simulink model "playback_data_example"  (R2016a)
settings: Solver=FixedStepDiscrete  SolverMode=SingleTasking  StartTime=76  StopTime=110  FixedStep=sample_time  RelTol=1e-3
values from neighbouring files (symbols this model uses):
  sample_time = 0.0005    [ElmoIncremental.m]
undefined symbols (not defined in the file or in its folder): control_start_time
libraries: simulink x1
settings Model: Creator=wmartin  LastModifiedBy=wmartin
settings SolverCC: EnableConcurrentExecution=on
settings DataIOCC: MaxDataPoints=1000000000  SaveFormat=StructureWithTime  SignalLogging=off  DSMLogging=off  VisualizeSimOutput=off
settings OptimizationCC: BlockReduction=off  OptimizeBlockIOStorage=off  BufferReuse=off  GlobalBufferReuse=off  ExpressionFolding=off  ExpressionDepthLimit=2147483647  LocalBlockOutputs=off  SimCompilerOptimization=on
settings DebuggingCC: UnderspecifiedInitializationDetection=Classic  MergeDetectMultiDrivingBlocksExec=none  SolverPrmCheckMsg=warning  StateNameClashWarn=warning
settings HardwareCC: ProdBitPerPointer=32  ProdLargestAtomicFloat=None  ProdWordSize=32  ProdLongLongMode=on  ProdHWDeviceType=Generic->32-bit x86 compatible
settings ModelReferenceCC: UpdateModelReferenceTargets=IfOutOfDate  ModelReferenceNumInstancesAllowed=Single  ModelReferenceMinAlgLoopOccurrences=on  PropagateSignalLabelsOutOfModel=off
settings RTWCC: SystemTargetFile=slrt.tlc  TemplateMakefile=slrt_default_tmf  Description=Simulink Real-Time  RTWVerbose=off  RTWCompilerOptimization=on
settings CodeAppCC: MaxIdLength=256
settings TargetCC: CodeReplacementLibrary=XPC_BLAS  ParMdlRefBuildCompliant=on  ConcurrentExecutionCompliant=on  MatFileLogging=on  MATLABClassNameForMDSCustomization=xpcAperiodicCustomization
settings ConfigComp: CovModelRefEnable=Off  CovSFcnEnable=off

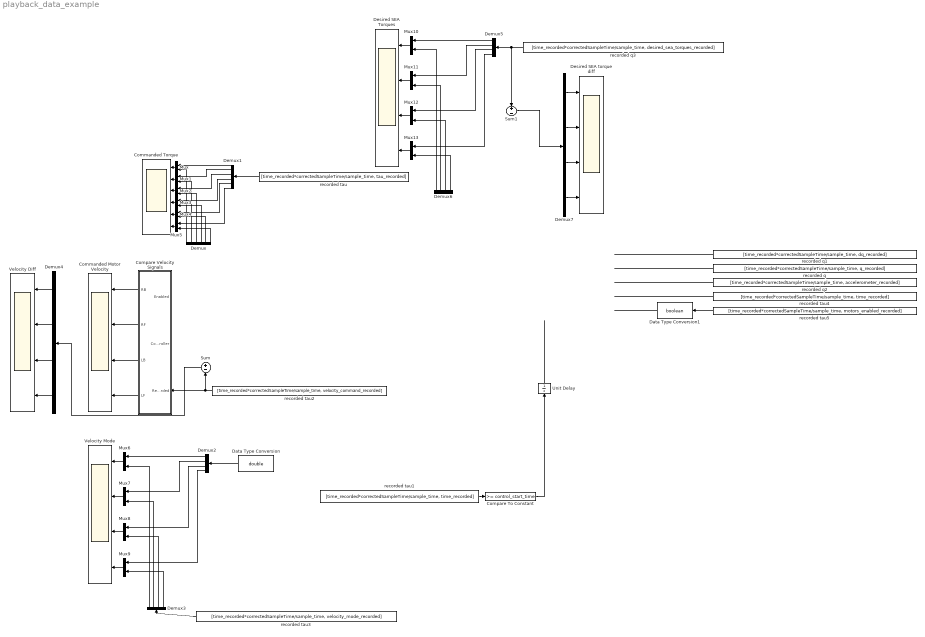
== system playback_data_example ==
  Commanded Motor Velocity : Scope  NumInputPorts=4
  Commanded Torque : Scope  NumInputPorts=6
  Compare To Constant : simulink/Logic and Bit Operations/Compare To Constant  relop=>=  const=control_start_time  OutDataTypeStr=boolean
  Compare Velocity Signals : Subsystem
  Data Type Conversion : DataTypeConversion  OutDataTypeStr=double
  Data Type Conversion1 : DataTypeConversion  OutDataTypeStr=boolean
  Demux : Demux  Outputs=6
  Demux1 : Demux  Outputs=6
  Demux{2..7} (6 alike) : Demux
  Desired SEA Torques : Scope  NumInputPorts=4
  Desired SEA torque diff : Scope  NumInputPorts=4
  Mux{,1..13} (14 alike) : Mux  Inputs=2
  Sum : Sum  Inputs=+-
  Sum1 : Sum  Inputs=+-
  Unit Delay : UnitDelay  SampleTime=-1
  Velocity Diff : Scope  NumInputPorts=4
  Velocity Mode : Scope  NumInputPorts=4
  recorded q : FromWorkspace  VariableName=[time_recorded*correctedSampleTime/sample_time, q_recorded]  OutDataTypeStr=double  SampleTime=sample_time  OutputAfterFinalValue=Holding final value
  recorded q1 : FromWorkspace  VariableName=[time_recorded*correctedSampleTime/sample_time, dq_recorded]  OutDataTypeStr=double  SampleTime=sample_time  OutputAfterFinalValue=Holding final value
  recorded q2 : FromWorkspace  VariableName=[time_recorded*correctedSampleTime/sample_time, accelerometer_recorded]  OutDataTypeStr=double  SampleTime=sample_time  OutputAfterFinalValue=Holding final value
  recorded q3 : FromWorkspace  VariableName=[time_recorded*correctedSampleTime/sample_time, desired_sea_torques_recorded]  OutDataTypeStr=double  SampleTime=sample_time  OutputAfterFinalValue=Holding final value
  recorded tau : FromWorkspace  VariableName=[time_recorded*correctedSampleTime/sample_time, tau_recorded]  OutDataTypeStr=double  SampleTime=sample_time  Interpolate=off  OutputAfterFinalValue=Holding final value
  recorded tau1 : FromWorkspace  VariableName=[time_recorded*correctedSampleTime/sample_time, time_recorded]  OutDataTypeStr=double  SampleTime=sample_time  OutputAfterFinalValue=Holding final value
  recorded tau2 : FromWorkspace  VariableName=[time_recorded*correctedSampleTime/sample_time, velocity_command_recorded]  OutDataTypeStr=double  SampleTime=sample_time  Interpolate=off  OutputAfterFinalValue=Holding final value
  recorded tau3 : FromWorkspace  VariableName=[time_recorded*correctedSampleTime/sample_time, velocity_mode_recorded]  OutDataTypeStr=double  SampleTime=sample_time  Interpolate=off  OutputAfterFinalValue=Holding final value
  recorded tau4 : FromWorkspace  VariableName=[time_recorded*correctedSampleTime/sample_time, time_recorded]  OutDataTypeStr=double  SampleTime=sample_time  OutputAfterFinalValue=Holding final value
  recorded tau5 : FromWorkspace  VariableName=[time_recorded*correctedSampleTime/sample_time, motors_enabled_recorded]  OutDataTypeStr=double  SampleTime=sample_time  OutputAfterFinalValue=Holding final value
  wires:
  recorded tau1/1 -> Compare To Constant/1
  Compare To Constant/1 -> Unit Delay/1
  Unit Delay/1 -> ?
  ? -> Demux/1
  recorded tau/1 -> Demux1/1
  Mux/1 -> Commanded Torque/1
  Mux1/1 -> Commanded Torque/2
  Mux2/1 -> Commanded Torque/3
  Mux3/1 -> Commanded Torque/4
  Mux4/1 -> Commanded Torque/5
  Mux5/1 -> Commanded Torque/6
  Demux1/1 -> Mux/1
  Demux/1 -> Mux/2
  Demux1/2 -> Mux1/1
  Demux1/3 -> Mux2/1
  Demux1/4 -> Mux3/1
  Demux1/5 -> Mux4/1
  Demux1/6 -> Mux5/1
  Demux/2 -> Mux1/2
  Demux/3 -> Mux2/2
  Demux/4 -> Mux3/2
  Demux/5 -> Mux4/2
  Demux/6 -> Mux5/2
  Compare Velocity Signals/1(RB) -> Commanded Motor Velocity/1
  Compare Velocity Signals/2(RF) -> Commanded Motor Velocity/2
  Compare Velocity Signals/3(LB) -> Commanded Motor Velocity/3
  Compare Velocity Signals/4(LF) -> Commanded Motor Velocity/4
  ? -> Compare Velocity Signals/1(Enabled), Data Type Conversion/1
  recorded tau2/1 -> Sum/2, Compare Velocity Signals/3(Recorded)
  Mux6/1 -> Velocity Mode/1
  Mux7/1 -> Velocity Mode/2
  Mux8/1 -> Velocity Mode/3
  Mux9/1 -> Velocity Mode/4
  Demux2/2 -> Mux7/1
  Demux2/3 -> Mux8/1
  Demux2/4 -> Mux9/1
  recorded tau3/1 -> Demux3/1
  Demux3/1 -> Mux6/2
  Demux3/2 -> Mux7/2
  Demux3/3 -> Mux8/2
  Demux3/4 -> Mux9/2
  Data Type Conversion/1 -> Demux2/1
  Demux2/1 -> Mux6/1
  ? -> Sum/1, Compare Velocity Signals/2(Controller)
  Sum/1 -> Demux4/1
  Demux4/4 -> Velocity Diff/4
  Demux4/3 -> Velocity Diff/3
  Demux4/2 -> Velocity Diff/2
  Demux4/1 -> Velocity Diff/1
  Mux10/1 -> Desired SEA Torques/1
  Mux11/1 -> Desired SEA Torques/2
  Mux12/1 -> Desired SEA Torques/3
  Mux13/1 -> Desired SEA Torques/4
  Demux5/2 -> Mux11/1
  Demux5/3 -> Mux12/1
  Demux5/4 -> Mux13/1
  Demux6/1 -> Mux10/2
  Demux6/2 -> Mux11/2
  Demux6/3 -> Mux12/2
  Demux6/4 -> Mux13/2
  recorded q3/1 -> Demux5/1, Sum1/1
  Demux5/1 -> Mux10/1
  ? -> Sum1/2, Demux6/1
  Demux7/3 -> Desired SEA torque diff/3
  Demux7/2 -> Desired SEA torque diff/2
  Demux7/1 -> Desired SEA torque diff/1
  Demux7/4 -> Desired SEA torque diff/4
  Sum1/1 -> Demux7/1
  recorded q1/1 -> ?
  recorded q/1 -> ?
  recorded q2/1 -> ?
  recorded tau4/1 -> ?
  Data Type Conversion1/1 -> ?
  recorded tau5/1 -> Data Type Conversion1/1

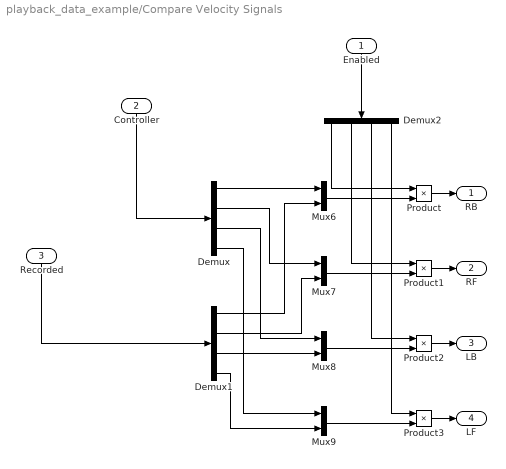
== system playback_data_example/Compare Velocity Signals ==
  Enabled : Inport
  Controller : Inport  Port=2
  Recorded : Inport  Port=3
  Demux : Demux
  Demux1 : Demux
  Demux2 : Demux
  Mux{6..9} (4 alike) : Mux  Inputs=2
  Product{,1..3} (4 alike) : Product
  RB : Outport
  RF : Outport  Port=2
  LB : Outport  Port=3
  LF : Outport  Port=4
  wires:
  Demux/3 -> Mux8/1
  Demux/2 -> Mux7/1
  Demux1/1 -> Mux6/2
  Demux/1 -> Mux6/1
  Product/1 -> RB/1
  Demux/4 -> Mux9/1
  Mux6/1 -> Product/2
  Demux1/4 -> Mux9/2
  Mux7/1 -> Product1/2
  Mux9/1 -> Product3/2
  Recorded/1 -> Demux1/1
  Demux2/3 -> Product2/1
  Demux1/2 -> Mux7/2
  Controller/1 -> Demux/1
  Demux2/1 -> Product/1
  Product3/1 -> LF/1
  Product1/1 -> RF/1
  Product2/1 -> LB/1
  Mux8/1 -> Product2/2
  Demux1/3 -> Mux8/2
  Enabled/1 -> Demux2/1
  Demux2/4 -> Product3/1
  Demux2/2 -> Product1/1
